simulink model "maglev_model"  (R2021a)
settings: Solver=ode4  StartTime=0.0  StopTime=10.0  FixedStep=0.001  RelTol=1e-3
values from neighbouring files (symbols this model uses):
  g = 9.81    [config_maglev.m]
  Km = 6.5308e-5    (= 6.5308e-05)    [config_maglev.m]
  Mb = 0.068    [config_maglev.m]
  Tb = 0.014    [config_maglev.m]
settings Model: Creator=MLevis  LastModifiedBy=MLevis

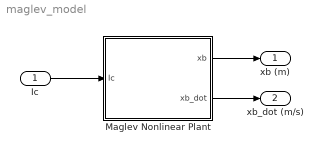
== system maglev_model ==
  Ic : Inport
  Maglev Nonlinear Plant : Subsystem
  xb (m) : Outport
  xb_dot (m/s) : Outport  Port=2
  wires:
  Ic/1 -> Maglev Nonlinear Plant/1(Ic)
  Maglev Nonlinear Plant/2(xb_dot) -> xb_dot (m/s)/1
  Maglev Nonlinear Plant/1(xb) -> xb (m)/1

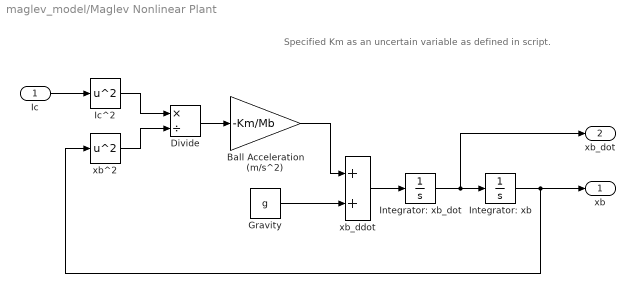
== system maglev_model/Maglev Nonlinear Plant ==
  note: Specified Km as an uncertain variable as defined in script.
  Ic : Inport
  Ball Acceleration (m/s^2) : Gain  SCDEnableBlockLinearizationSpecification=on  Gain=-Km/Mb
  Divide : Product  Inputs=*/
  Gravity : Constant  Value=g
  Ic^2 : Math  Operator=square  SignedPower=on  SaturateOnIntegerOverflow=on
  Integrator: xb : Integrator  InitialCondition=Tb  LimitOutput=on  UpperSaturationLimit=Tb  LowerSaturationLimit=0
  Integrator: xb_dot : Integrator
  xb^2 : Math  Operator=square  SignedPower=on  SaturateOnIntegerOverflow=on
  xb_ddot : Sum
  xb : Outport
  xb_dot : Outport  Port=2
  wires:
  Gravity/1 -> xb_ddot/2
  xb_ddot/1 -> Integrator: xb_dot/1
  Integrator: xb_dot/1 -> xb_dot/1, Integrator: xb/1
  Divide/1 -> Ball Acceleration (m/s^2)/1
  Ball Acceleration (m/s^2)/1 -> xb_ddot/1
  xb^2/1 -> Divide/2
  Ic^2/1 -> Divide/1
  Integrator: xb/1 -> xb/1, xb^2/1
  Ic/1 -> Ic^2/1
